simulink model "HEV"  (R2015a)
settings: Solver=ode23tb  StartTime=0.0  StopTime=318  FixedStep=Ts  MaxStep=Ts  RelTol=1  AbsTol=0.5
InitFcn:
  | Ts = 6e-05;   % time step
  | DriveCycleNumber = 1;
  | beginningSim = 1;
undefined symbols (not defined in the file): drive_block, drive_enginemodel, EngineSpeedPower, FuelConsTable, GasEmisTable, h, Hydride, km, magnitude, Metal, Nickel, rad, s, speed, torque
libraries: powerlib x47, driveline x30, simulink x13, simulink_extras x9, electricdrivelib x3, powerlib_extras x3, aerolibconvert2 x2, DC6DriveInternalModels x1
(part 2 of 3)

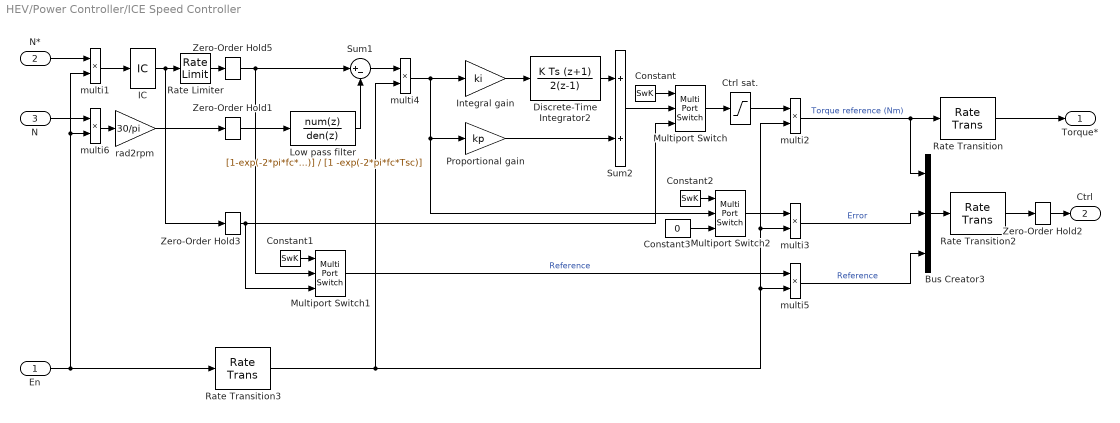
== system HEV/Power Controller/ICE Speed Controller ==
  En : Inport
  N* : Inport  Port=2
  N : Inport  Port=3
  Bus Creator3 : BusCreator  Inputs=3
  Constant : Constant  Value=SwK
  Constant1 : Constant  Value=SwK
  Constant2 : Constant  Value=SwK
  Constant3 : Constant  Value=0
  Ctrl sat. : Saturate  UpperLimit=ctrl_sat(2)  LowerLimit=ctrl_sat(1)
  Discrete-Time Integrator2 : DiscreteIntegrator  IntegratorMethod=Integration: Trapezoidal  SampleTime=Tsc  LimitOutput=on  UpperSaturationLimit=ctrl_sat(2)  LowerSaturationLimit=ctrl_sat(1)
  IC : InitialCondition  Value=0
  Integral gain : Gain  Gain=ki  SaturateOnIntegerOverflow=on  OutDataTypeStr=Inherit: Same as input  ParamDataTypeStr=Inherit: Same as input
  Low pass filter : DiscreteTransferFcn  Numerator=[1-exp(-2*pi*fc*Tsc)]  Denominator=[1 -exp(-2*pi*fc*Tsc)]  SampleTime=Tsc
  Multiport Switch : MultiPortSwitch  Inputs=2  SaturateOnIntegerOverflow=on
  Multiport Switch1 : MultiPortSwitch  Inputs=2  SaturateOnIntegerOverflow=on
  Multiport Switch2 : MultiPortSwitch  Inputs=2  SaturateOnIntegerOverflow=on
  Proportional gain : Gain  Gain=kp  SaturateOnIntegerOverflow=on  OutDataTypeStr=Inherit: Same as input  ParamDataTypeStr=Inherit: Same as input
  Rate Limiter : RateLimiter  RisingSlewLimit=ramp(2)  FallingSlewLimit=ramp(1)  LinearizeAsGain=off
  Rate Transition : RateTransition
  Rate Transition2 : RateTransition
  Rate Transition3 : RateTransition
  Sum1 : Sum  Inputs=|+-  SaturateOnIntegerOverflow=on  InputSameDT=on  OutDataTypeStr=Inherit: Same as first input
  Sum2 : Sum  SaturateOnIntegerOverflow=on  InputSameDT=on  OutDataTypeStr=Inherit: Same as first input
  Zero-Order Hold1 : ZeroOrderHold  SampleTime=Tsc
  Zero-Order Hold2 : ZeroOrderHold  SampleTime=Ts
  Zero-Order Hold3 : ZeroOrderHold  SampleTime=Tsc
  Zero-Order Hold5 : ZeroOrderHold  SampleTime=Tsc
  multi{1..6} (6 alike) : Product
  rad2rpm : Gain  Gain=30/pi  SaturateOnIntegerOverflow=on  OutDataTypeStr=Inherit: Same as input  ParamDataTypeStr=Inherit: Same as input
  Torque* : Outport
  Ctrl : Outport  Port=2
  wires:
  N/1 -> multi6/1
  multi6/1 -> rad2rpm/1
  N*/1 -> multi1/1
  multi1/1 -> IC/1
  Rate Transition3/1 -> multi5/2, multi2/2, multi3/2, multi4/2
  multi4/1 -> Proportional gain/1, Multiport Switch2/2, Integral gain/1
  Low pass filter/1 -> Sum1/2
  multi2/1 -> Bus Creator3/1, Rate Transition/1  "Torque reference (Nm)"
  Multiport Switch1/1 -> multi5/1  "Reference"
  multi5/1 -> Bus Creator3/3  "Reference"
  multi3/1 -> Bus Creator3/2  "Error"
  Multiport Switch2/1 -> multi3/1
  Zero-Order Hold2/1 -> Ctrl/1
  Rate Transition/1 -> Torque*/1
  En/1 -> multi6/2, multi1/2, Rate Transition3/1
  rad2rpm/1 -> Zero-Order Hold1/1
  Constant3/1 -> Multiport Switch2/3
  Constant2/1 -> Multiport Switch2/1
  Zero-Order Hold3/1 -> Multiport Switch1/3, Multiport Switch/3
  Constant1/1 -> Multiport Switch1/1
  Sum2/1 -> Multiport Switch/2
  Constant/1 -> Multiport Switch/1
  Multiport Switch/1 -> Ctrl sat./1
  Zero-Order Hold5/1 -> Multiport Switch1/2, Sum1/1
  Rate Limiter/1 -> Zero-Order Hold5/1
  Bus Creator3/1 -> Rate Transition2/1
  Rate Transition2/1 -> Zero-Order Hold2/1
  Zero-Order Hold1/1 -> Low pass filter/1
  IC/1 -> Zero-Order Hold3/1, Rate Limiter/1
  Proportional gain/1 -> Sum2/2
  Discrete-Time Integrator2/1 -> Sum2/1
  Sum1/1 -> multi4/1
  Integral gain/1 -> Discrete-Time Integrator2/1
  Ctrl sat./1 -> multi2/1

== system HEV/Power Controller/Limit torque ==
  Acceleration : Inport
  Motor Speed (rad/s) : Inport  Port=2
  Abs1 : Abs  SaturateOnIntegerOverflow=on
  Clock1 : Clock
  Compare To Constant : simulink/Logic and Bit Operations/Compare To Constant  relop=>  const=0.05  OutDataTypeStr=uint8  ZeroCross=off
  Gain : Gain  Gain=-1
  Max Torque : Gain  Gain=400
  Product : Product  RndMeth=Zero
  Saturation Dynamic : simulink/Discontinuities/Saturation Dynamic  OutMin=[]  OutMax=[]  OutDataTypeStr=Inherit: Same as second input  OutDataType=sfix(16)  OutScaling=2^-10  DoSatur=off
  Torque vs speed : Lookup  InputValues=[0 1200 2000 3000 4000 5000 6000]*pi/30  Table=[400 400 225 150 100 80 70]  LookUpMeth=Interpolation-Use End Values
  torque : Outport
  wires:
  Motor Speed (rad/s)/1 -> Abs1/1
  Abs1/1 -> Torque vs speed/1
  Max Torque/1 -> Saturation Dynamic/2
  Torque vs speed/1 -> Gain/1, Saturation Dynamic/1
  Clock1/1 -> Compare To Constant/1
  Saturation Dynamic/1 -> Product/1
  Compare To Constant/1 -> Product/2
  Product/1 -> torque/1
  Gain/1 -> Saturation Dynamic/3
  Acceleration/1 -> Max Torque/1

== system HEV/Electric Motor Controller /DC//DC Converter/Bus DC controller ==
  Ubus : Inport
  Uref : Inport  Port=2
  Current controller DISCRETE1 : Subsystem  mask(PI controller){Kp=0.001, Ki=1, Ts=Ts}
      mask prompts: Kp "Proportional gain (Kp)"; Ki "Integral gain (Ki)"; Ts "Sample time (s) :"
      mask help: Proportional-Integral Speed Controller
      mask Display: plot(0,0,100,100,[35,35,65],[70,30,30],[35,65],[45,60])
  Display : Display
      settings: Decimation=100
  Duty Cycles : Subsystem
  Mux : Mux  Inputs=2
  Unit Delay2 : UnitDelay  InitialCondition=.5  SampleTime=Ts
  Zero-Order Hold1 : ZeroOrderHold  SampleTime=Ts
  Duty cycle : Outport  InitialOutput=0
  tag scope: V_DCDC=global
  wires:
  Ubus/1 -> Mux/2, Zero-Order Hold1/1
  Mux/1 -> [V_DCDC]
  Uref/1 -> Current controller DISCRETE1/2(Uref), Mux/1
  Current controller DISCRETE1/1(Ec) -> Duty Cycles/1(Ec)
  Zero-Order Hold1/1 -> Display/1, Current controller DISCRETE1/1(UBus)
  Duty Cycles/1(dc) -> Unit Delay2/1
  Unit Delay2/1 -> Duty cycle/1

== system HEV/Electric Motor Controller /DC//DC Converter/DC//DC converter ==
  Duty Cycle : Inport
  CBus : powerlib/Elements/Series RLC Branch  LConnTagsString=__new0  RConnTagsString=__new0  BranchType=RC  Resistance=0.2  Inductance=1e-3  SetiL0=off  InitialCurrent=0  Capacitance=1130e-6  Setx0=on  InitialVoltage=500  Measurements=None
  CBus1 : powerlib/Elements/Series RLC Branch  LConnTagsString=__new0  RConnTagsString=__new0  BranchType=C  Resistance=0.2  Inductance=1e-3  SetiL0=off  InitialCurrent=0  Capacitance=282e-6  Setx0=on  InitialVoltage=150  Measurements=None
  Chopper : DC6DriveInternalModels/Chopper (average model)  SnubberResistance=10e3  SnubberCapacitance=inf  Ron=1e-3  ForwardVoltages=[1.3,1.3]  IGBTParameters=[0,0]  converterType=Inverter
  L : powerlib/Elements/Series RLC Branch  LConnTagsString=__new0  RConnTagsString=__new0  BranchType=L  Resistance=0.3  Inductance=373e-6  SetiL0=off  InitialCurrent=100  Capacitance=100e-6  Setx0=off  InitialVoltage=0  Measurements=None
  Neutral2 : powerlib/Elements/Neutral  LConnTagsString=a  NodeNumber=10
  V1 : powerlib/Measurements/Voltage Measurement  PhasorSimulation=off  OutputType=Complex  PSBequivalent=0
  + : PMIOPort  Tag=PMCPort  Port=1  Side=Left
  - : PMIOPort  Tag=PMCPort  Port=2  Side=Left
  + bat. : PMIOPort  Tag=PMCPort  Port=3  Side=Right
  - bat. : PMIOPort  Tag=PMCPort  Port=4  Side=Right
  UBus : Outport
  wires:
  Duty Cycle/1 -> Chopper/1
  V1/1 -> UBus/1
  connections:
  Chopper/RConn1 -- L/RConn1
  L/LConn1 -- + bat./RConn1 -- CBus1/LConn1
  CBus1/RConn1 -- - bat./RConn1 -- Chopper/LConn2 -- -/RConn1 -- CBus/RConn1 -- V1/LConn2 -- Neutral2/LConn1
  +/RConn1 -- CBus/LConn1 -- Chopper/LConn1 -- V1/LConn1

== system HEV/Electric Motor Controller /Generator 30kW/Mux ==
  sig* : Inport
  m : Inport  Port=2
  Bus Creator : BusCreator  Inputs=2
  Ctrl : Outport
  wires:
  m/1 -> Bus Creator/2  "m"
  sig*/1 -> Bus Creator/1  "Signals*"
  Bus Creator/1 -> Ctrl/1

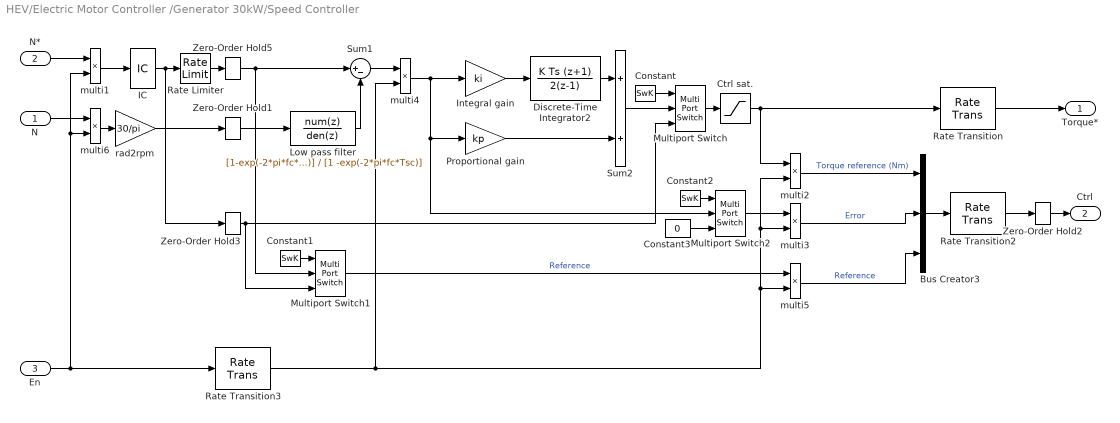
== system HEV/Electric Motor Controller /Generator 30kW/Speed Controller ==
  N : Inport
  N* : Inport  Port=2
  En : Inport  Port=3
  Bus Creator3 : BusCreator  Inputs=3
  Constant : Constant  Value=SwK
  Constant1 : Constant  Value=SwK
  Constant2 : Constant  Value=SwK
  Constant3 : Constant  Value=0
  Ctrl sat. : Saturate  UpperLimit=ctrl_sat(2)  LowerLimit=ctrl_sat(1)
  Discrete-Time Integrator2 : DiscreteIntegrator  IntegratorMethod=Integration: Trapezoidal  SampleTime=Tsc  LimitOutput=on  UpperSaturationLimit=ctrl_sat(2)  LowerSaturationLimit=ctrl_sat(1)
  IC : InitialCondition  Value=0
  Integral gain : Gain  Gain=ki  SaturateOnIntegerOverflow=on  OutDataTypeStr=Inherit: Same as input  ParamDataTypeStr=Inherit: Same as input
  Low pass filter : DiscreteTransferFcn  Numerator=[1-exp(-2*pi*fc*Tsc)]  Denominator=[1 -exp(-2*pi*fc*Tsc)]  SampleTime=Tsc
  Multiport Switch : MultiPortSwitch  Inputs=2  SaturateOnIntegerOverflow=on
  Multiport Switch1 : MultiPortSwitch  Inputs=2  SaturateOnIntegerOverflow=on
  Multiport Switch2 : MultiPortSwitch  Inputs=2  SaturateOnIntegerOverflow=on
  Proportional gain : Gain  Gain=kp  SaturateOnIntegerOverflow=on  OutDataTypeStr=Inherit: Same as input  ParamDataTypeStr=Inherit: Same as input
  Rate Limiter : RateLimiter  RisingSlewLimit=ramp(2)  FallingSlewLimit=ramp(1)  LinearizeAsGain=off
  Rate Transition : RateTransition
  Rate Transition2 : RateTransition
  Rate Transition3 : RateTransition
  Sum1 : Sum  Inputs=|+-  SaturateOnIntegerOverflow=on  InputSameDT=on  OutDataTypeStr=Inherit: Same as first input
  Sum2 : Sum  SaturateOnIntegerOverflow=on  InputSameDT=on  OutDataTypeStr=Inherit: Same as first input
  Zero-Order Hold1 : ZeroOrderHold  SampleTime=Tsc
  Zero-Order Hold2 : ZeroOrderHold  SampleTime=Ts
  Zero-Order Hold3 : ZeroOrderHold  SampleTime=Tsc
  Zero-Order Hold5 : ZeroOrderHold  SampleTime=Tsc
  multi{1..6} (6 alike) : Product
  rad2rpm : Gain  Gain=30/pi  SaturateOnIntegerOverflow=on  OutDataTypeStr=Inherit: Same as input  ParamDataTypeStr=Inherit: Same as input
  Torque* : Outport
  Ctrl : Outport  Port=2
  wires:
  N/1 -> multi6/1
  multi6/1 -> rad2rpm/1
  N*/1 -> multi1/1
  multi1/1 -> IC/1
  Rate Transition3/1 -> multi5/2, multi2/2, multi3/2, multi4/2
  multi4/1 -> Multiport Switch2/2, Proportional gain/1, Integral gain/1
  Low pass filter/1 -> Sum1/2
  multi2/1 -> Bus Creator3/1  "Torque reference (Nm)"
  Multiport Switch1/1 -> multi5/1  "Reference"
  multi5/1 -> Bus Creator3/3  "Reference"
  multi3/1 -> Bus Creator3/2  "Error"
  Multiport Switch2/1 -> multi3/1
  Zero-Order Hold2/1 -> Ctrl/1
  Rate Transition/1 -> Torque*/1
  En/1 -> multi6/2, multi1/2, Rate Transition3/1
  rad2rpm/1 -> Zero-Order Hold1/1
  Constant3/1 -> Multiport Switch2/3
  Constant2/1 -> Multiport Switch2/1
  Zero-Order Hold3/1 -> Multiport Switch1/3, Multiport Switch/3
  Constant1/1 -> Multiport Switch1/1
  Sum2/1 -> Multiport Switch/2
  Constant/1 -> Multiport Switch/1
  Multiport Switch/1 -> Ctrl sat./1
  Zero-Order Hold5/1 -> Multiport Switch1/2, Sum1/1
  Rate Limiter/1 -> Zero-Order Hold5/1
  Bus Creator3/1 -> Rate Transition2/1
  Rate Transition2/1 -> Zero-Order Hold2/1
  Zero-Order Hold1/1 -> Low pass filter/1
  IC/1 -> Zero-Order Hold3/1, Rate Limiter/1
  Proportional gain/1 -> Sum2/2
  Discrete-Time Integrator2/1 -> Sum2/1
  Sum1/1 -> multi4/1
  Integral gain/1 -> Discrete-Time Integrator2/1
  Ctrl sat./1 -> multi2/1, Rate Transition/1

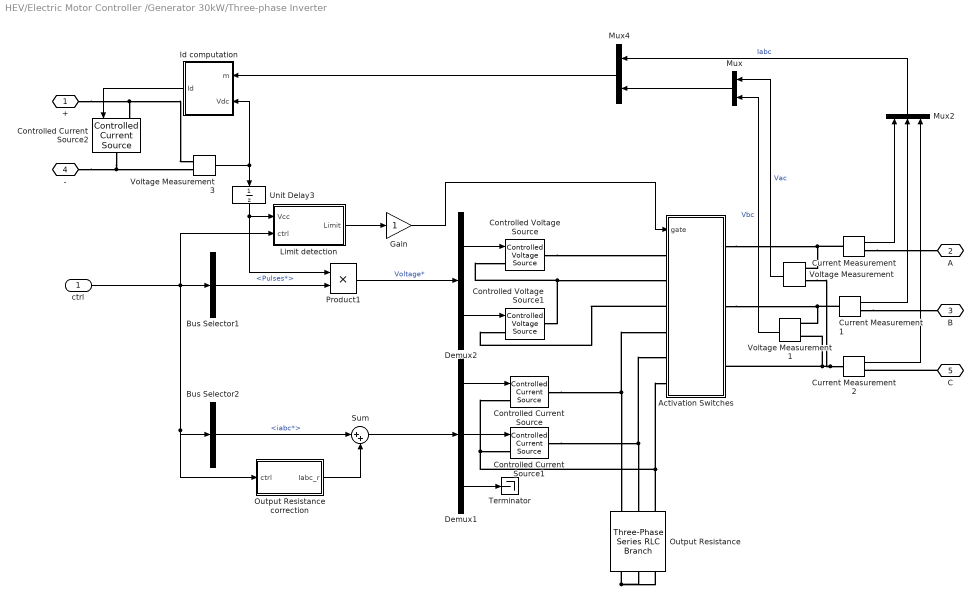
== system HEV/Electric Motor Controller /Generator 30kW/Three-phase Inverter ==
  ctrl : Inport
  Activation Switches : Subsystem
  Bus Selector1 : BusSelector  OutputSignals=Signals*.Pulses*
  Bus Selector2 : BusSelector  OutputSignals=Signals*.iabc*
  Controlled Current Source : powerlib/Electrical Sources/Controlled Current Source  Initialize=on  Source_Type=AC  Amplitude=0  Phase=0  Frequency=0  Measurements=None
  Controlled Current Source1 : powerlib/Electrical Sources/Controlled Current Source  Initialize=on  Source_Type=AC  Amplitude=0  Phase=0  Frequency=0  Measurements=None
  Controlled Current Source2 : powerlib/Electrical Sources/Controlled Current Source  Initialize=on  Source_Type=AC  Amplitude=0  Phase=0  Frequency=0  Measurements=None
  Controlled Voltage Source : powerlib/Electrical Sources/Controlled Voltage Source  Initialize=on  Source_Type=AC  Amplitude=0  Phase=0  Frequency=0  Measurements=None
  Controlled Voltage Source1 : powerlib/Electrical Sources/Controlled Voltage Source  Initialize=on  Source_Type=AC  Amplitude=0  Phase=0  Frequency=0  Measurements=None
  Current Measurement : powerlib/Measurements/Current Measurement  PhasorSimulation=off  OutputType=Complex  PSBequivalent=0
  Current Measurement1 : powerlib/Measurements/Current Measurement  PhasorSimulation=off  OutputType=Complex  PSBequivalent=0
  Current Measurement2 : powerlib/Measurements/Current Measurement  PhasorSimulation=off  OutputType=Complex  PSBequivalent=0
  Demux1 : Demux  Outputs=3
  Demux2 : Demux  Outputs=2
  Gain : Gain
  Id computation : Subsystem
  Limit detection : Subsystem
  Mux : Mux  Inputs=2
  Mux2 : Mux  Inputs=3
  Mux4 : Mux  Inputs=2
  Output Resistance : powerlib/Elements/Three-Phase Series RLC Branch  LConnTagsString=A|B|C  RConnTagsString=A|B|C  BranchType=R  Resistance=100*Resistance  Inductance=1e-3  Capacitance=1e-6  Measurements=Branch voltages and currents
  Output Resistance correction : Subsystem
  Product1 : Product  RndMeth=Zero
  Sum : Sum  Inputs=|++
  Terminator : Terminator
  Unit Delay3 : UnitDelay  SampleTime=Ts
  Voltage Measurement : powerlib/Measurements/Voltage Measurement  PhasorSimulation=off  OutputType=Complex  PSBequivalent=0
  Voltage Measurement1 : powerlib/Measurements/Voltage Measurement  PhasorSimulation=off  OutputType=Complex  PSBequivalent=0
  Voltage Measurement3 : powerlib/Measurements/Voltage Measurement  PhasorSimulation=off  OutputType=Complex  PSBequivalent=0
  + : PMIOPort  Port=1  Side=Right
  A : PMIOPort  Port=2  Side=Left
  B : PMIOPort  Port=3  Side=Left
  - : PMIOPort  Port=4  Side=Right
  C : PMIOPort  Port=5  Side=Left
  wires:
  Gain/1 -> Activation Switches/1(gate)
  Output Resistance correction/1("Iabc_r ") -> Sum/2
  Product1/1 -> Demux2/1  "Voltage*"
  ctrl/1 -> Output Resistance correction/1(ctrl), Bus Selector2/1, Limit detection/2(ctrl), Bus Selector1/1
  Unit Delay3/1 -> Limit detection/1(Vcc), Product1/1
  Sum/1 -> Demux1/1
  Limit detection/1(Limit) -> Gain/1
  Bus Selector2/1 -> Sum/1  "<iabc*>"
  Demux2/1 -> Controlled Voltage Source/1
  Demux2/2 -> Controlled Voltage Source1/1
  Demux1/3 -> Terminator/1
  Demux1/2 -> Controlled Current Source1/1
  Demux1/1 -> Controlled Current Source/1
  Bus Selector1/1 -> Product1/2  "<Pulses*>"
  Voltage Measurement3/1 -> Id computation/2(Vdc), Unit Delay3/1
  Id computation/1(Id) -> Controlled Current Source2/1
  Mux2/1 -> Mux4/1  "Iabc"
  Mux4/1 -> Id computation/1(m)
  Current Measurement2/1 -> Mux2/3
  Mux/1 -> Mux4/2
  Voltage Measurement1/1 -> Mux/2  "Vbc"
  Voltage Measurement/1 -> Mux/1  "Vac"
  Current Measurement1/1 -> Mux2/2
  Current Measurement/1 -> Mux2/1
  connections:
  Activation Switches/LConn3 -- Controlled Voltage Source1/LConn1
  Controlled Voltage Source/RConn1 -- Activation Switches/LConn1
  C/RConn1 -- Current Measurement2/RConn1
  Current Measurement1/RConn1 -- B/RConn1
  Current Measurement/RConn1 -- A/RConn1
  Current Measurement1/LConn1 -- Activation Switches/RConn2 -- Voltage Measurement1/LConn1
  Controlled Voltage Source1/RConn1 -- Activation Switches/LConn2 -- Controlled Voltage Source/LConn1
  Current Measurement2/LConn1 -- Voltage Measurement1/LConn2 -- Activation Switches/RConn3 -- Voltage Measurement/LConn2
  Controlled Current Source1/RConn1 -- Activation Switches/LConn5 -- Output Resistance/LConn2
  Controlled Current Source/RConn1 -- Activation Switches/LConn4 -- Output Resistance/LConn1
  Current Measurement/LConn1 -- Activation Switches/RConn1 -- Voltage Measurement/LConn1
  Output Resistance/RConn1 -- Output Resistance/RConn2 -- Output Resistance/RConn3
  Output Resistance/LConn3 -- Controlled Current Source1/LConn1 -- Controlled Current Source/LConn1 -- Activation Switches/LConn6
  -/RConn1 -- Controlled Current Source2/RConn1 -- Voltage Measurement3/LConn2
  +/RConn1 -- Controlled Current Source2/LConn1 -- Voltage Measurement3/LConn1

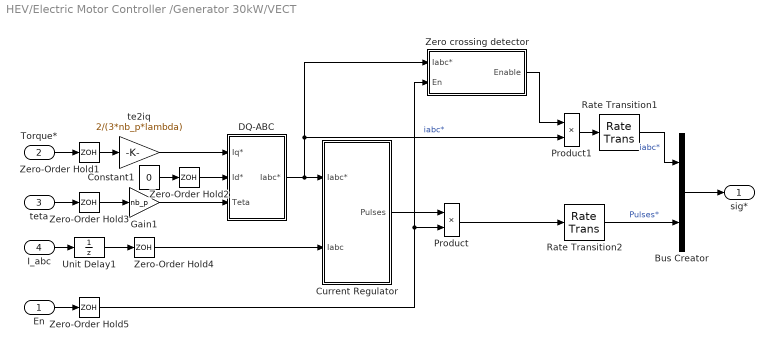
== system HEV/Electric Motor Controller /Generator 30kW/VECT ==
  En : Inport
  Torque* : Inport  Port=2
  teta : Inport  Port=3
  I_abc : Inport  Port=4
  Bus Creator : BusCreator  Inputs=2
  Constant1 : Constant  Value=0
  Current Regulator : Subsystem
  DQ-ABC : Subsystem
  Gain1 : Gain  Gain=nb_p  SaturateOnIntegerOverflow=on  OutDataTypeStr=Inherit: Same as input  ParamDataTypeStr=Inherit: Same as input
  Product : Product  RndMeth=Zero
  Product1 : Product  RndMeth=Zero
  Rate Transition1 : RateTransition
  Rate Transition2 : RateTransition
  Unit Delay1 : UnitDelay  SampleTime=Ts
  Zero crossing detector : Subsystem
  Zero-Order Hold{1..5} (5 alike) : ZeroOrderHold  SampleTime=Ts_vect
  te2iq : Gain  Gain=2/(3*nb_p*lambda)  SaturateOnIntegerOverflow=on  OutDataTypeStr=Inherit: Same as input  ParamDataTypeStr=Inherit: Same as input
  sig* : Outport
  wires:
  Zero-Order Hold5/1 -> Zero crossing detector/2(En), Product/2
  Zero crossing detector/1(Enable) -> Product1/1
  En/1 -> Zero-Order Hold5/1
  Product1/1 -> Rate Transition1/1
  Product/1 -> Rate Transition2/1
  Current Regulator/1(Pulses) -> Product/1
  Zero-Order Hold4/1 -> Current Regulator/2(Iabc)
  Rate Transition1/1 -> Bus Creator/1  "iabc*"
  Rate Transition2/1 -> Bus Creator/2  "Pulses*"
  Bus Creator/1 -> sig*/1
  te2iq/1 -> DQ-ABC/1("Iq* ")
  Zero-Order Hold2/1 -> DQ-ABC/2("Id* ")
  Zero-Order Hold1/1 -> te2iq/1
  teta/1 -> Zero-Order Hold3/1
  Zero-Order Hold3/1 -> Gain1/1
  Torque*/1 -> Zero-Order Hold1/1
  Constant1/1 -> Zero-Order Hold2/1
  Gain1/1 -> DQ-ABC/3(Teta)
  Unit Delay1/1 -> Zero-Order Hold4/1
  DQ-ABC/1(Iabc*) -> Zero crossing detector/1(Iabc*), Product1/2, Current Regulator/1(Iabc*)  "iabc*"
  I_abc/1 -> Unit Delay1/1

== system HEV/Electric Motor Controller /Motor 50kW/Mux ==
  sig : Inport
  m : Inport  Port=2
  Bus Creator : BusCreator  Inputs=2
  Ctrl : Outport
  wires:
  Bus Creator/1 -> Ctrl/1
  sig/1 -> Bus Creator/1  "sig"
  m/1 -> Bus Creator/2  "m"

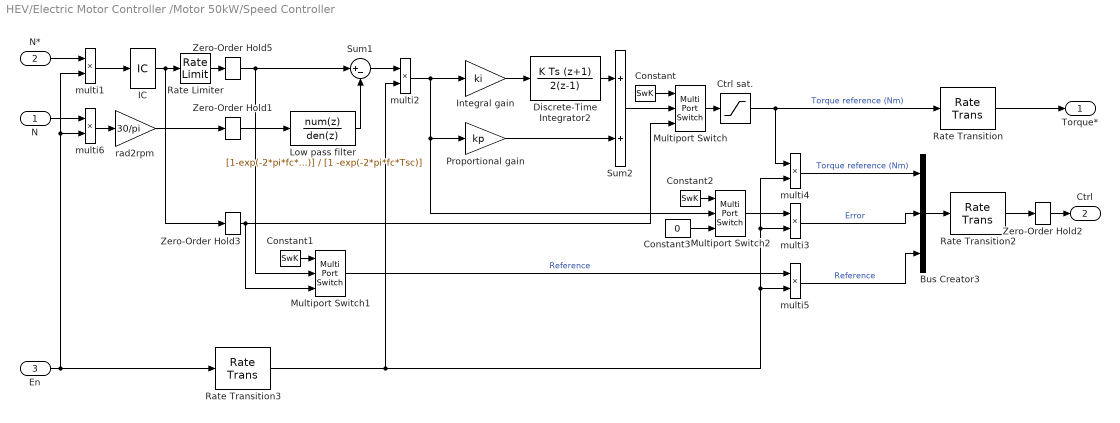
== system HEV/Electric Motor Controller /Motor 50kW/Speed Controller ==
  N : Inport
  N* : Inport  Port=2
  En : Inport  Port=3
  Bus Creator3 : BusCreator  Inputs=3
  Constant : Constant  Value=SwK
  Constant1 : Constant  Value=SwK
  Constant2 : Constant  Value=SwK
  Constant3 : Constant  Value=0
  Ctrl sat. : Saturate  UpperLimit=ctrl_sat(2)  LowerLimit=ctrl_sat(1)
  Discrete-Time Integrator2 : DiscreteIntegrator  IntegratorMethod=Integration: Trapezoidal  SampleTime=Tsc  LimitOutput=on  UpperSaturationLimit=ctrl_sat(2)  LowerSaturationLimit=ctrl_sat(1)
  IC : InitialCondition  Value=0
  Integral gain : Gain  Gain=ki  SaturateOnIntegerOverflow=on  OutDataTypeStr=Inherit: Same as input  ParamDataTypeStr=Inherit: Same as input
  Low pass filter : DiscreteTransferFcn  Numerator=[1-exp(-2*pi*fc*Tsc)]  Denominator=[1 -exp(-2*pi*fc*Tsc)]  SampleTime=Tsc
  Multiport Switch : MultiPortSwitch  Inputs=2  SaturateOnIntegerOverflow=on
  Multiport Switch1 : MultiPortSwitch  Inputs=2  SaturateOnIntegerOverflow=on
  Multiport Switch2 : MultiPortSwitch  Inputs=2  SaturateOnIntegerOverflow=on
  Proportional gain : Gain  Gain=kp  SaturateOnIntegerOverflow=on  OutDataTypeStr=Inherit: Same as input  ParamDataTypeStr=Inherit: Same as input
  Rate Limiter : RateLimiter  RisingSlewLimit=ramp(2)  FallingSlewLimit=ramp(1)  LinearizeAsGain=off
  Rate Transition : RateTransition
  Rate Transition2 : RateTransition
  Rate Transition3 : RateTransition
  Sum1 : Sum  Inputs=|+-  SaturateOnIntegerOverflow=on  InputSameDT=on  OutDataTypeStr=Inherit: Same as first input
  Sum2 : Sum  SaturateOnIntegerOverflow=on  InputSameDT=on  OutDataTypeStr=Inherit: Same as first input
  Zero-Order Hold1 : ZeroOrderHold  SampleTime=Tsc
  Zero-Order Hold2 : ZeroOrderHold  SampleTime=Ts
  Zero-Order Hold3 : ZeroOrderHold  SampleTime=Tsc
  Zero-Order Hold5 : ZeroOrderHold  SampleTime=Tsc
  multi{1..6} (6 alike) : Product
  rad2rpm : Gain  Gain=30/pi  SaturateOnIntegerOverflow=on  OutDataTypeStr=Inherit: Same as input  ParamDataTypeStr=Inherit: Same as input
  Torque* : Outport
  Ctrl : Outport  Port=2
  wires:
  Ctrl sat./1 -> multi4/1, Rate Transition/1  "Torque reference (Nm)"
  Integral gain/1 -> Discrete-Time Integrator2/1
  Sum1/1 -> multi2/1
  Discrete-Time Integrator2/1 -> Sum2/1
  Proportional gain/1 -> Sum2/2
  IC/1 -> Rate Limiter/1, Zero-Order Hold3/1
  Zero-Order Hold1/1 -> Low pass filter/1
  Rate Transition2/1 -> Zero-Order Hold2/1
  Bus Creator3/1 -> Rate Transition2/1
  Low pass filter/1 -> Sum1/2
  Rate Limiter/1 -> Zero-Order Hold5/1
  Zero-Order Hold5/1 -> Sum1/1, Multiport Switch1/2
  Multiport Switch/1 -> Ctrl sat./1
  Constant/1 -> Multiport Switch/1
  Sum2/1 -> Multiport Switch/2
  Constant1/1 -> Multiport Switch1/1
  Zero-Order Hold3/1 -> Multiport Switch/3, Multiport Switch1/3
  Constant2/1 -> Multiport Switch2/1
  Constant3/1 -> Multiport Switch2/3
  rad2rpm/1 -> Zero-Order Hold1/1
  En/1 -> Rate Transition3/1, multi1/2, multi6/2
  Rate Transition/1 -> Torque*/1
  Zero-Order Hold2/1 -> Ctrl/1
  Multiport Switch2/1 -> multi3/1
  multi3/1 -> Bus Creator3/2  "Error"
  multi5/1 -> Bus Creator3/3  "Reference"
  Multiport Switch1/1 -> multi5/1  "Reference"
  multi4/1 -> Bus Creator3/1  "Torque reference (Nm)"
  multi2/1 -> Integral gain/1, Proportional gain/1, Multiport Switch2/2
  Rate Transition3/1 -> multi2/2, multi4/2, multi3/2, multi5/2
  multi6/1 -> rad2rpm/1
  multi1/1 -> IC/1
  N*/1 -> multi1/1
  N/1 -> multi6/1

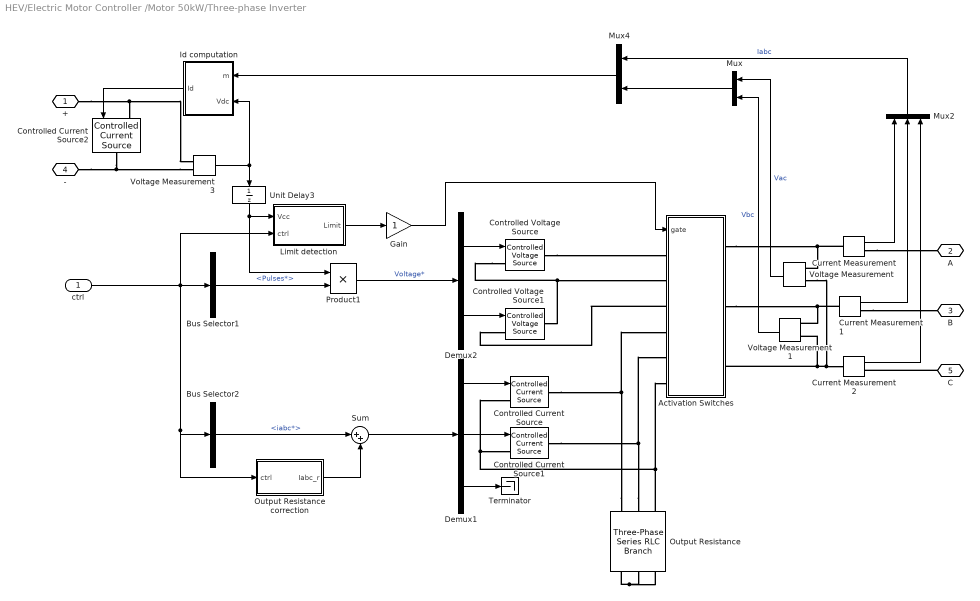
== system HEV/Electric Motor Controller /Motor 50kW/Three-phase Inverter ==
  ctrl : Inport
  Activation Switches : Subsystem
  Bus Selector1 : BusSelector  OutputSignals=sig.Pulses*
  Bus Selector2 : BusSelector  OutputSignals=sig.iabc*
  Controlled Current Source : powerlib/Electrical Sources/Controlled Current Source  Initialize=on  Source_Type=AC  Amplitude=0  Phase=0  Frequency=0  Measurements=None
  Controlled Current Source1 : powerlib/Electrical Sources/Controlled Current Source  Initialize=on  Source_Type=AC  Amplitude=0  Phase=0  Frequency=0  Measurements=None
  Controlled Current Source2 : powerlib/Electrical Sources/Controlled Current Source  Initialize=on  Source_Type=AC  Amplitude=0  Phase=0  Frequency=0  Measurements=None
  Controlled Voltage Source : powerlib/Electrical Sources/Controlled Voltage Source  Initialize=on  Source_Type=AC  Amplitude=0  Phase=0  Frequency=0  Measurements=None
  Controlled Voltage Source1 : powerlib/Electrical Sources/Controlled Voltage Source  Initialize=on  Source_Type=AC  Amplitude=0  Phase=0  Frequency=0  Measurements=None
  Current Measurement : powerlib/Measurements/Current Measurement  PhasorSimulation=off  OutputType=Complex  PSBequivalent=0
  Current Measurement1 : powerlib/Measurements/Current Measurement  PhasorSimulation=off  OutputType=Complex  PSBequivalent=0
  Current Measurement2 : powerlib/Measurements/Current Measurement  PhasorSimulation=off  OutputType=Complex  PSBequivalent=0
  Demux1 : Demux  Outputs=3
  Demux2 : Demux  Outputs=2
  Gain : Gain
  Id computation : Subsystem
  Limit detection : Subsystem
  Mux : Mux  Inputs=2
  Mux2 : Mux  Inputs=3
  Mux4 : Mux  Inputs=2
  Output Resistance : powerlib/Elements/Three-Phase Series RLC Branch  LConnTagsString=A|B|C  RConnTagsString=A|B|C  BranchType=R  Resistance=100*Resistance  Inductance=1e-3  Capacitance=1e-6  Measurements=Branch voltages and currents
  Output Resistance correction : Subsystem
  Product1 : Product  RndMeth=Zero
  Sum : Sum  Inputs=|++
  Terminator : Terminator
  Unit Delay3 : UnitDelay  SampleTime=Ts
  Voltage Measurement : powerlib/Measurements/Voltage Measurement  PhasorSimulation=off  OutputType=Complex  PSBequivalent=0
  Voltage Measurement1 : powerlib/Measurements/Voltage Measurement  PhasorSimulation=off  OutputType=Complex  PSBequivalent=0
  Voltage Measurement3 : powerlib/Measurements/Voltage Measurement  PhasorSimulation=off  OutputType=Complex  PSBequivalent=0
  + : PMIOPort  Port=1  Side=Right
  A : PMIOPort  Port=2  Side=Left
  B : PMIOPort  Port=3  Side=Left
  - : PMIOPort  Port=4  Side=Right
  C : PMIOPort  Port=5  Side=Left
  wires:
  Current Measurement/1 -> Mux2/1
  Current Measurement1/1 -> Mux2/2
  Voltage Measurement/1 -> Mux/1  "Vac"
  Voltage Measurement1/1 -> Mux/2  "Vbc"
  Mux/1 -> Mux4/2
  Current Measurement2/1 -> Mux2/3
  Mux4/1 -> Id computation/1(m)
  Mux2/1 -> Mux4/1  "Iabc"
  Voltage Measurement3/1 -> Unit Delay3/1, Id computation/2(Vdc)
  Bus Selector1/1 -> Product1/2  "<Pulses*>"
  Demux1/1 -> Controlled Current Source/1
  Demux1/2 -> Controlled Current Source1/1
  Demux1/3 -> Terminator/1
  Demux2/2 -> Controlled Voltage Source1/1
  Demux2/1 -> Controlled Voltage Source/1
  Bus Selector2/1 -> Sum/1  "<iabc*>"
  Limit detection/1(Limit) -> Gain/1
  Sum/1 -> Demux1/1
  Unit Delay3/1 -> Product1/1, Limit detection/1(Vcc)
  ctrl/1 -> Bus Selector1/1, Limit detection/2(ctrl), Bus Selector2/1, Output Resistance correction/1(ctrl)
  Product1/1 -> Demux2/1  "Voltage*"
  Gain/1 -> Activation Switches/1(gate)
  Id computation/1(Id) -> Controlled Current Source2/1
  Output Resistance correction/1("Iabc_r ") -> Sum/2
  connections:
  Voltage Measurement3/LConn1 -- Controlled Current Source2/LConn1 -- +/RConn1
  Voltage Measurement3/LConn2 -- Controlled Current Source2/RConn1 -- -/RConn1
  Activation Switches/LConn6 -- Controlled Current Source/LConn1 -- Controlled Current Source1/LConn1 -- Output Resistance/LConn3
  Output Resistance/RConn3 -- Output Resistance/RConn2 -- Output Resistance/RConn1
  Voltage Measurement/LConn1 -- Activation Switches/RConn1 -- Current Measurement/LConn1
  Output Resistance/LConn1 -- Activation Switches/LConn4 -- Controlled Current Source/RConn1
  Output Resistance/LConn2 -- Activation Switches/LConn5 -- Controlled Current Source1/RConn1
  Voltage Measurement/LConn2 -- Activation Switches/RConn3 -- Voltage Measurement1/LConn2 -- Current Measurement2/LConn1
  Controlled Voltage Source/LConn1 -- Activation Switches/LConn2 -- Controlled Voltage Source1/RConn1
  Voltage Measurement1/LConn1 -- Activation Switches/RConn2 -- Current Measurement1/LConn1
  Current Measurement/RConn1 -- A/RConn1
  Current Measurement1/RConn1 -- B/RConn1
  C/RConn1 -- Current Measurement2/RConn1
  Controlled Voltage Source/RConn1 -- Activation Switches/LConn1
  Activation Switches/LConn3 -- Controlled Voltage Source1/LConn1

== system HEV/Electric Motor Controller /Motor 50kW/Torque limitation ==
  N rad/s : Inport
  Torque : Inport  Port=2
  Abs1 : Abs  SaturateOnIntegerOverflow=on
  Gain : Gain  Gain=-1
  Saturation Dynamic : simulink/Discontinuities/Saturation Dynamic  OutMin=[]  OutMax=[]  OutDataTypeStr=Inherit: Same as second input  OutDataType=sfix(16)  OutScaling=2^-10  DoSatur=off
  Torque vs speed profile : Lookup  InputValues=[0 1200 2000 3000 4000 5000 6000]*pi/30  Table=[400 400 225 150 100 80 70]  LookUpMeth=Interpolation-Use End Values
  torque : Outport
  wires:
  N rad/s/1 -> Abs1/1
  Abs1/1 -> Torque vs speed profile/1
  Torque vs speed profile/1 -> Saturation Dynamic/1, Gain/1
  Saturation Dynamic/1 -> torque/1
  Torque/1 -> Saturation Dynamic/2
  Gain/1 -> Saturation Dynamic/3

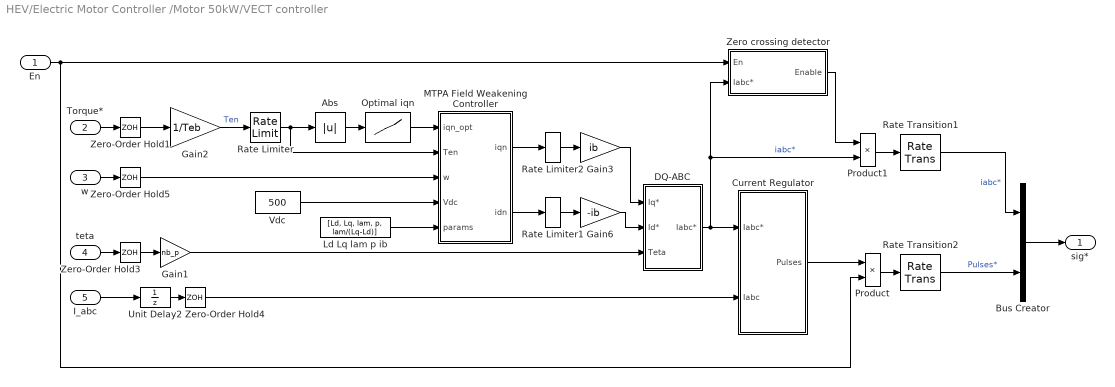
== system HEV/Electric Motor Controller /Motor 50kW/VECT controller ==
  En : Inport
  Torque* : Inport  Port=2
  w : Inport  Port=3
  teta : Inport  Port=4
  I_abc : Inport  Port=5
  Abs : Abs
  Bus Creator : BusCreator  Inputs=2
  Current Regulator : Subsystem
  DQ-ABC : Subsystem
  Gain1 : Gain  Gain=nb_p  SaturateOnIntegerOverflow=on  OutDataTypeStr=Inherit: Same as input  ParamDataTypeStr=Inherit: Same as input
  Gain2 : Gain  Gain=1/Teb  SaturateOnIntegerOverflow=on  OutDataTypeStr=Inherit: Same as input  ParamDataTypeStr=Inherit: Same as input
  Gain3 : Gain  Gain=ib  SaturateOnIntegerOverflow=on  OutDataTypeStr=Inherit: Same as input  ParamDataTypeStr=Inherit: Same as input
  Gain6 : Gain  Gain=-ib  SaturateOnIntegerOverflow=on  OutDataTypeStr=Inherit: Same as input  ParamDataTypeStr=Inherit: Same as input
  Ld Lq lam p ib : Constant  Value=[Ld, Lq, lam, p, lam/(Lq-Ld)]
  MTPA Field Weakening Controller : MATLAB Function  TreatAsAtomicUnit=on  SystemSampleTime=Ts_vect
  Optimal iqn : Lookup  InputValues=ten  Table=iqn
  Product : Product  RndMeth=Zero
  Product1 : Product  RndMeth=Zero
  Rate Limiter : RateLimiter  RisingSlewLimit=10  FallingSlewLimit=-10  LinearizeAsGain=off
  Rate Limiter1 : RateLimiter  RisingSlewLimit=100  FallingSlewLimit=-100  SampleTimeMode=inherited
  Rate Limiter2 : RateLimiter  RisingSlewLimit=100  FallingSlewLimit=-100  SampleTimeMode=inherited
  Rate Transition1 : RateTransition
  Rate Transition2 : RateTransition
  Unit Delay2 : UnitDelay  SampleTime=-1
  Vdc : Constant  Value=500
  Zero crossing detector : Subsystem
  Zero-Order Hold{1,3..5} (4 alike) : ZeroOrderHold  SampleTime=Ts_vect
  sig* : Outport
  wires:
  Unit Delay2/1 -> Zero-Order Hold4/1
  Zero-Order Hold4/1 -> Current Regulator/2(Iabc)
  teta/1 -> Zero-Order Hold3/1
  Zero-Order Hold3/1 -> Gain1/1
  Gain1/1 -> DQ-ABC/3(Teta)
  DQ-ABC/1(Iabc*) -> Current Regulator/1(Iabc*), Zero crossing detector/2(Iabc*), Product1/2  "iabc*"
  I_abc/1 -> Unit Delay2/1
  Torque*/1 -> Zero-Order Hold1/1
  Gain3/1 -> DQ-ABC/1("Iq* ")
  Gain6/1 -> DQ-ABC/2("Id* ")
  Zero-Order Hold1/1 -> Gain2/1
  w/1 -> Zero-Order Hold5/1
  MTPA Field Weakening Controller/2(idn) -> Rate Limiter1/1
  Gain2/1 -> Rate Limiter/1  "Ten"
  Zero-Order Hold5/1 -> MTPA Field Weakening Controller/3(w)
  Ld Lq lam p ib/1 -> MTPA Field Weakening Controller/5(params)
  MTPA Field Weakening Controller/1(iqn) -> Rate Limiter2/1
  Optimal iqn/1 -> MTPA Field Weakening Controller/1(iqn_opt)
  Abs/1 -> Optimal iqn/1
  Vdc/1 -> MTPA Field Weakening Controller/4(Vdc)
  Bus Creator/1 -> sig*/1
  Rate Transition2/1 -> Bus Creator/2  "Pulses*"
  Rate Transition1/1 -> Bus Creator/1  "iabc*"
  Current Regulator/1(Pulses) -> Product/1
  Product/1 -> Rate Transition2/1
  Product1/1 -> Rate Transition1/1
  Zero crossing detector/1(Enable) -> Product1/1
  En/1 -> Zero crossing detector/1(En), Product/2
  Rate Limiter2/1 -> Gain3/1
  Rate Limiter1/1 -> Gain6/1
  Rate Limiter/1 -> Abs/1, MTPA Field Weakening Controller/2(Ten)

== system HEV/Engine Controller/Fuel and Gas Emissions Calculation/Fuel Conversion ==
  Vehicle Speed (km/h) : Inport
  Fuel Consumption (g/s) : Inport  Port=2
  Divide : Product  Inputs=*/
  Gasoline density kg/m^3 : Constant  Value=719.7
  Integrator (total km) : Integrator  InitialCondition=eps
  Integrator (total l) : Integrator  InitialCondition=eps
  Reciprocal : Math  Operator=reciprocal  SaturateOnIntegerOverflow=on
  Saturation : Saturate  UpperLimit=Inf  LowerLimit=0
  Saturation1 : Saturate  UpperLimit=Inf  LowerLimit=0
  Saturation2 : Saturate  UpperLimit=Inf  LowerLimit=0
  Velocity Conversion : aerolibconvert2/Velocity Conversion  IU=km/h  OU=km/s
  g/s to kg/s : Gain  Gain=0.001
  l/km to l/100km : Gain  Gain=100
  liters per km : Product  Inputs=/*
  m^3 to liters : Gain  Gain=1000
  l/100km : Outport
  km/l : Outport  Port=2
  Total Fuel (l) : Outport  Port=3
  wires:
  Vehicle Speed (km/h)/1 -> Velocity Conversion/1
  Velocity Conversion/1 -> Integrator (total km)/1
  Fuel Consumption (g/s)/1 -> g/s to kg/s/1
  g/s to kg/s/1 -> Divide/1
  Gasoline density kg/m^3/1 -> Divide/2
  Divide/1 -> m^3 to liters/1
  m^3 to liters/1 -> Integrator (total l)/1
  Integrator (total km)/1 -> liters per km/1
  Integrator (total l)/1 -> Saturation/1, liters per km/2
  liters per km/1 -> Reciprocal/1, l/km to l/100km/1
  l/km to l/100km/1 -> Saturation2/1
  Reciprocal/1 -> Saturation1/1
  Saturation/1 -> Total Fuel (l)/1
  Saturation1/1 -> km/l/1
  Saturation2/1 -> l/100km/1

== system HEV/Power Controller/Game Theory Controller/Battery Available Power ==
  T ICE : Inport
  P* ICE : Inport  Port=2
  Battery recharge : Inport  Port=3
  ICE speed (rad/s) : Inport  Port=4
  Power limit : Inport  Port=5
  Add2 : Sum  Inputs=-+
  Compare To Zero : simulink/Logic and Bit Operations/Compare To Zero  relop=~=  OutDataTypeStr=boolean
  Gain : Gain  Gain=-1
  Multiplication1 : Product
  Multiplication2 : Product
  Mux2 : Mux  Inputs=2
  Rate Limiter : RateLimiter  RisingSlewLimit=21e3  FallingSlewLimit=-21e3  SampleTimeMode=inherited
  Relay2 : Relay  OnSwitchValue=12e3  OffSwitchValue=11e3
  Saturation Dynamic : simulink/Discontinuities/Saturation Dynamic  OutMin=[]  OutMax=[]  OutDataTypeStr=Inherit: Same as second input  OutDataType=sfix(16)  OutScaling=2^-10  DoSatur=off
  Switch1 : Switch  Criteria=u2 ~= 0
  Switch2 : Switch  Criteria=u2 ~= 0
  Battery power : Outport
  "ICE (P*, P)" : Outport  Port=2
  wires:
  ICE speed (rad/s)/1 -> Multiplication1/2
  Saturation Dynamic/1 -> Battery power/1
  P* ICE/1 -> Add2/2, Multiplication2/1, Relay2/1
  Power limit/1 -> Gain/1, Saturation Dynamic/1
  Gain/1 -> Saturation Dynamic/3
  Mux2/1 -> "ICE (P*, P)"/1
  Relay2/1 -> Multiplication2/2
  Multiplication2/1 -> Mux2/1
  T ICE/1 -> Multiplication1/1
  Multiplication1/1 -> Add2/1, Mux2/2  "P ICE"
  Battery recharge/1 -> Switch1/1, Compare To Zero/1
  Compare To Zero/1 -> Switch1/2, Switch2/2
  Add2/1 -> Switch1/3, Switch2/3  "P batt"
  Switch1/1 -> Rate Limiter/1
  Rate Limiter/1 -> Switch2/1
  Switch2/1 -> Saturation Dynamic/2

== system HEV/Power Controller/Game Theory Controller/Gen torque ==
  T* ICE : Inport
  W gen : Inport  Port=2
  " 1" : Gain  Gain=-1
  " 3" : Gain  Gain=30e3
  " 4" : Gain  Gain=-1/(-2.6-1)
  Abs1 : Abs
  Gen Torque range : simulink/Discontinuities/Saturation Dynamic  OutMin=[]  OutMax=[]  OutDataTypeStr=Inherit: Same as second input  OutDataType=sfix(16)  OutScaling=2^-10  DoSatur=off
  Multiplication2 : Product  Inputs=/
  zero avoider1 : Saturate  UpperLimit=inf  LowerLimit=1
  T* Gen : Outport
  wires:
  T* ICE/1 -> " 4"/1
  Multiplication2/1 -> " 3"/1
  " 3"/1 -> Abs1/1
  W gen/1 -> zero avoider1/1
  Abs1/1 -> Gen Torque range/1, " 1"/1
  " 1"/1 -> Gen Torque range/3
  " 4"/1 -> Gen Torque range/2
  Gen Torque range/1 -> T* Gen/1
  zero avoider1/1 -> Multiplication2/1

== system HEV/Power Controller/Game Theory Controller/Hybrid On//Off ==
  Ref Power : Inport
  Recharge power : Inport  Port=2
  Compare To Zero : simulink/Logic and Bit Operations/Compare To Zero  relop=~=  OutDataTypeStr=boolean
  Compare To Zero1 : simulink/Logic and Bit Operations/Compare To Zero  relop=>  OutDataTypeStr=boolean
  Logical Operator1 : Logic  Operator=OR  AllPortsSameDT=off  OutDataTypeStr=boolean
  Logical Operator2 : Logic  Operator=NOT  AllPortsSameDT=off  OutDataTypeStr=boolean
  Logical Operator3 : Logic  AllPortsSameDT=off  OutDataTypeStr=boolean
  Memory : Memory
  Relay2 : Relay  OnSwitchValue=12e3  OffSwitchValue=11e3  OnOutputValue=0  OffOutputValue=1
  Hybrid : Outport
  wires:
  Relay2/1 -> Logical Operator2/1
  Memory/1 -> Compare To Zero/1
  Logical Operator2/1 -> Logical Operator1/1
  Compare To Zero/1 -> Logical Operator3/2
  Logical Operator3/1 -> Logical Operator1/2
  Compare To Zero1/1 -> Logical Operator3/1
  Ref Power/1 -> Relay2/1, Compare To Zero1/1
  Recharge power/1 -> Memory/1
  Logical Operator1/1 -> Hybrid/1  "Hybrid"

== system HEV/Power Controller/Game Theory Controller/ICE Torque ==
  note: This subsystem is used to calculate the ICE required torque.
      | Also, it calculates the torques needed to stop the ICE when the hybrid mode is off.
  Hybrid : Inport
  W gen : Inport  Port=2
  w* ICE (rpm) : Inport  Port=3
  P* ICE : Inport  Port=4
  w ICE (rad/s) : Inport  Port=5
  ICE Power range : Saturate  UpperLimit=57e3  LowerLimit=-57e3
  Multiplication1 : Product
  Multiplication2 : Product  Inputs=3
  Multiplication3 : Product  Inputs=/*
  Multiplication5 : Product  Inputs=/*
  Rate Limiter2 : RateLimiter  RisingSlewLimit=10  FallingSlewLimit=-10
  Relay1 : Relay  OnSwitchValue=300  OffSwitchValue=200
  Sample & Hold : powerlib_extras/Control  Blocks/Sample & Hold  ic=0
  rpm2rads : Gain  Gain=pi/30
  shed limit : Saturate  UpperLimit=1  LowerLimit=0
  T* ICE : Outport
  wires:
  Relay1/1 -> Rate Limiter2/1
  Hybrid/1 -> Sample & Hold/2
  P* ICE/1 -> ICE Power range/1
  w* ICE (rpm)/1 -> rpm2rads/1
  Multiplication5/1 -> Multiplication1/2  "T* ICE"
  Multiplication1/1 -> Sample & Hold/1
  Multiplication2/1 -> T* ICE/1
  Rate Limiter2/1 -> Multiplication1/1, Multiplication2/1
  ICE Power range/1 -> Multiplication5/2
  rpm2rads/1 -> Multiplication5/1, Multiplication3/1
  w ICE (rad/s)/1 -> Multiplication3/2
  Multiplication3/1 -> shed limit/1  "Loadshed if w < w*"
  Sample & Hold/1 -> Multiplication2/2
  shed limit/1 -> Multiplication2/3
  W gen/1 -> Relay1/1

== system HEV/Electric Motor Controller /DC//DC Converter/Bus DC controller/Current controller DISCRETE1 ==
  UBus : Inport
  Uref : Inport  Port=2
  Clock1 : Clock
  Compare To Constant1 : simulink/Logic and Bit Operations/Compare To Constant  relop=>  const=0.01  OutDataTypeStr=uint8  ZeroCross=off
  Ctrl sat. : Saturate  UpperLimit=0.95  LowerLimit=-0.95
  Discrete-Time Integrator : DiscreteIntegrator  IntegratorMethod=Integration: Trapezoidal  SampleTime=Ts  LimitOutput=on  UpperSaturationLimit=1  LowerSaturationLimit=-1
  Integral gain : Gain  Gain=Ki  SaturateOnIntegerOverflow=on  OutDataTypeStr=Inherit: Same as input  ParamDataTypeStr=Inherit: Same as input
  Product1 : Product  RndMeth=Zero
  Proportional gain : Gain  Gain=Kp  SaturateOnIntegerOverflow=on  OutDataTypeStr=Inherit: Same as input  ParamDataTypeStr=Inherit: Same as input
  Sum1 : Sum  Inputs=+-  SaturateOnIntegerOverflow=on  InputSameDT=on  OutDataTypeStr=Inherit: Same as first input
  Sum2 : Sum  SaturateOnIntegerOverflow=on  InputSameDT=on  OutDataTypeStr=Inherit: Same as first input
  Ec : Outport  InitialOutput=0
  wires:
  Sum2/1 -> Ctrl sat./1
  Discrete-Time Integrator/1 -> Sum2/2
  Uref/1 -> Sum1/2
  UBus/1 -> Sum1/1
  Integral gain/1 -> Discrete-Time Integrator/1
  Proportional gain/1 -> Sum2/1
  Ctrl sat./1 -> Ec/1
  Sum1/1 -> Product1/1
  Clock1/1 -> Compare To Constant1/1
  Compare To Constant1/1 -> Product1/2
  Product1/1 -> Integral gain/1, Proportional gain/1

== system HEV/Electric Motor Controller /DC//DC Converter/Bus DC controller/Duty Cycles ==
  Ec : Inport
  Add : Sum  Inputs=+-
  Bus Creator2 : BusCreator  Inputs=2
  Constant : Constant
  Duty Cycle : Fcn  Expr=0.5*(u[1]+1)
  dc : Outport
  wires:
  Bus Creator2/1 -> dc/1
  Ec/1 -> Duty Cycle/1
  Constant/1 -> Add/1
  Add/1 -> Bus Creator2/2  "IGBT 2"
  Duty Cycle/1 -> Bus Creator2/1, Add/2  "IGBT I"

== system HEV/Electric Motor Controller /Generator 30kW/Three-phase Inverter/Activation Switches ==
  gate : Inport
  Ideal Switch1 : powerlib/Power Electronics/Ideal Switch  Ron=2*Ron  Lon=0  IC=1  Rs=1e6  Cs=inf  Measurements=off
  Ideal Switch2 : powerlib/Power Electronics/Ideal Switch  Ron=2*Ron  Lon=0  IC=1  Rs=1e6  Cs=inf  Measurements=off
  Ideal Switch3 : powerlib/Power Electronics/Ideal Switch  Ron=2*Ron  Lon=0  IC=1  Rs=1e6  Cs=inf  Measurements=off
  Ideal Switch4 : powerlib/Power Electronics/Ideal Switch  Ron=2*Ron  Lon=0  IC=0  Rs=1e6  Cs=inf  Measurements=off
  Ideal Switch5 : powerlib/Power Electronics/Ideal Switch  Ron=2*Ron  Lon=0  IC=0  Rs=1e6  Cs=inf  Measurements=off
  Ideal Switch6 : powerlib/Power Electronics/Ideal Switch  Ron=2*Ron  Lon=0  IC=0  Rs=1e6  Cs=inf  Measurements=off
  Logical Operator : Logic  Operator=NOT  AllPortsSameDT=off  OutDataTypeStr=boolean
  A1 : PMIOPort  Port=1  Side=Left
  a : PMIOPort  Port=2  Side=Right
  B1 : PMIOPort  Port=3  Side=Left
  b : PMIOPort  Port=4  Side=Right
  C1 : PMIOPort  Port=5  Side=Left
  c : PMIOPort  Port=6  Side=Right
  A2 : PMIOPort  Port=7  Side=Left
  B2 : PMIOPort  Port=8  Side=Left
  C2 : PMIOPort  Port=9  Side=Left
  wires:
  Logical Operator/1 -> Ideal Switch6/1, Ideal Switch5/1, Ideal Switch4/1
  gate/1 -> Logical Operator/1, Ideal Switch3/1, Ideal Switch2/1, Ideal Switch1/1
  connections:
  C2/RConn1 -- Ideal Switch6/LConn1
  B2/RConn1 -- Ideal Switch5/LConn1
  A2/RConn1 -- Ideal Switch4/LConn1
  c/RConn1 -- Ideal Switch6/RConn1 -- Ideal Switch3/RConn1
  C1/RConn1 -- Ideal Switch3/LConn1
  b/RConn1 -- Ideal Switch5/RConn1 -- Ideal Switch2/RConn1
  B1/RConn1 -- Ideal Switch2/LConn1
  Ideal Switch4/RConn1 -- a/RConn1 -- Ideal Switch1/RConn1
  A1/RConn1 -- Ideal Switch1/LConn1

== system HEV/Electric Motor Controller /Generator 30kW/Three-phase Inverter/Id computation ==
  m : Inport
  Vdc : Inport  Port=2
  Demux : Subsystem
  Demux1 : Subsystem
  Gain : Gain  Gain=Ron
  Math Function : Math  Operator=magnitude^2  SaturateOnIntegerOverflow=on
  Math Function1 : Math  Operator=magnitude^2  SaturateOnIntegerOverflow=on
  Math Function2 : Math  Operator=magnitude^2  SaturateOnIntegerOverflow=on
  Product1 : Product  Inputs=*/  SaturateOnIntegerOverflow=on  OutDataTypeStr=Inherit: Same as first input
  Sum1 : Sum  Inputs=+++  SaturateOnIntegerOverflow=on
  Sum2 : Sum  Inputs=|++  SaturateOnIntegerOverflow=on
  Sum3 : Sum  SaturateOnIntegerOverflow=on
  Unit Delay1 : UnitDelay  SampleTime=Ts
  Unit Delay4 : UnitDelay  InitialCondition=1  SampleTime=Ts
  Vac x Ia : Product  SaturateOnIntegerOverflow=on  OutDataTypeStr=Inherit: Same as first input
  Vbc x Ib : Product  SaturateOnIntegerOverflow=on  OutDataTypeStr=Inherit: Same as first input
  Zero avoider : Saturate  UpperLimit=inf  LowerLimit=1
  Id : Outport
  wires:
  Zero avoider/1 -> Product1/2
  Product1/1 -> Id/1
  Gain/1 -> Sum2/2
  Demux/3(Vbc) -> Vbc x Ib/1
  Demux/4(Ib) -> Vbc x Ib/2
  Demux/2(Ia) -> Vac x Ia/2
  Demux/1(Vac) -> Vac x Ia/1
  Vdc/1 -> Unit Delay4/1
  Vbc x Ib/1 -> Sum3/2
  Vac x Ia/1 -> Sum3/1
  m/1 -> Demux/1(m), Demux1/1(m)
  Unit Delay1/1 -> Product1/1
  Unit Delay4/1 -> Zero avoider/1
  Demux1/1(Ia) -> Math Function/1
  Demux1/2(Ib) -> Math Function1/1
  Demux1/3(Ic) -> Math Function2/1
  Math Function1/1 -> Sum1/2
  Math Function/1 -> Sum1/1
  Math Function2/1 -> Sum1/3
  Sum1/1 -> Gain/1
  Sum3/1 -> Sum2/1
  Sum2/1 -> Unit Delay1/1

== system HEV/Electric Motor Controller /Generator 30kW/Three-phase Inverter/Limit detection ==
  note: Low pass filter
  note: Low pass filter
  note: Limit = 1 saturation mode (voltage mode)
      | Limit = 0 normal mode (current mode)
  Vcc : Inport
  ctrl : Inport  Port=2
  Bus Selector1 : BusSelector  OutputSignals=m.Stator current is_d (A),m.Stator current is_q (A),m.Rotor speed wm (rad/s)  OutputAsBus=on
  Discrete Transfer Fcn1 : DiscreteTransferFcn  Numerator=[1-exp(-Ts*Fcs*2*pi)]  Denominator=[1 -exp(-Ts*Fcs*2*pi)]  SampleTime=Ts
  Discrete Transfer Fcn3 : DiscreteTransferFcn  Numerator=[1-exp(-Ts*Fcs*2*pi)]  Denominator=[1 -exp(-Ts*Fcs*2*pi)]  SampleTime=Ts
  Gain1 : Gain  Gain=0.9  SaturateOnIntegerOverflow=on  OutDataTypeStr=Inherit: Same as input  ParamDataTypeStr=Inherit: Same as input
  "Internal Vcc " : Fcn  Expr=pi/2*sqrt((Resistance*u(1)-Lq*p*u(3)*u(2))^2+(Resistance*u(2)+Ld*p*u(3)*u(1)+Flux*p*u(3))^2)
  Relational Operator : RelationalOperator  Operator=>  OutDataTypeStr=boolean
  Relational Operator2 : RelationalOperator  Operator=<  OutDataTypeStr=boolean
  S-R Flip-Flop : simulink_extras/Flip Flops/S-R Flip-Flop  initial_condition=0
  Terminator : Terminator
  Limit : Outport
  wires:
  S-R Flip-Flop/2 -> Terminator/1
  Discrete Transfer Fcn3/1 -> Relational Operator/2, Gain1/1
  Gain1/1 -> Relational Operator2/2
  Discrete Transfer Fcn1/1 -> Relational Operator2/1, Relational Operator/1
  "Internal Vcc "/1 -> Discrete Transfer Fcn1/1
  Bus Selector1/1 -> "Internal Vcc "/1
  ctrl/1 -> Bus Selector1/1
  S-R Flip-Flop/1 -> Limit/1
  Relational Operator2/1 -> S-R Flip-Flop/2
  Relational Operator/1 -> S-R Flip-Flop/1
  Vcc/1 -> Discrete Transfer Fcn3/1

== system HEV/Electric Motor Controller /Generator 30kW/Three-phase Inverter/Output Resistance correction ==
  note: Vabc
  ctrl : Inport
  1/R : Gain  Gain=1/(100*Resistance)  SaturateOnIntegerOverflow=on  OutDataTypeStr=Inherit: Same as input  ParamDataTypeStr=Inherit: Same as input
  Bus Selector1 : BusSelector  OutputSignals=m.Stator voltage Vs_d (V),m.Stator voltage Vs_q (V),m.Rotor angle thetam (rad)
  Constant : Constant  Value=0
  Discrete Transfer Fcn1 : DiscreteTransferFcn  Numerator=[1-exp(-Ts/.001)]  Denominator=[1 -exp(-Ts/.001)]  SampleTime=Ts
  Discrete Transfer Fcn2 : DiscreteTransferFcn  Numerator=[1-exp(-Ts/.001)]  Denominator=[1 -exp(-Ts/.001)]  SampleTime=Ts
  Fcn : Fcn  Expr=sin(u)
  Fcn1 : Fcn  Expr=cos(u)
  Mux4 : Mux  Inputs=3
  Mux5 : Mux  Inputs=2
  dq0_to_abc Transformation : powerlib_extras/Measurements/dq0_to_abc Transformation
  poles : Gain  Gain=p  SaturateOnIntegerOverflow=on  OutDataTypeStr=Inherit: Same as input  ParamDataTypeStr=Inherit: Same as input
  "Iabc_r " : Outport
  wires:
  poles/1 -> Fcn/1, Fcn1/1
  Bus Selector1/3 -> poles/1  "<Rotor angle thetam (rad)>"
  Discrete Transfer Fcn1/1 -> Mux4/1
  Discrete Transfer Fcn2/1 -> Mux4/2
  dq0_to_abc Transformation/1 -> 1/R/1
  Constant/1 -> Mux4/3
  Mux5/1 -> dq0_to_abc Transformation/2
  Fcn1/1 -> Mux5/2
  Fcn/1 -> Mux5/1
  Mux4/1 -> dq0_to_abc Transformation/1
  ctrl/1 -> Bus Selector1/1
  Bus Selector1/1 -> Discrete Transfer Fcn1/1  "<Stator voltage Vs_d (V)>"
  Bus Selector1/2 -> Discrete Transfer Fcn2/1  "<Stator voltage Vs_q (V)>"
  1/R/1 -> "Iabc_r "/1

== system HEV/Electric Motor Controller /Generator 30kW/VECT/Current Regulator ==
  Iabc* : Inport
  Iabc : Inport  Port=2
  Demux1 : Demux  Outputs=3
  Demux2 : Demux  Outputs=3
  Mux1 : Mux  Inputs=2
  Relay : Relay  OnSwitchValue=0  OffSwitchValue=0
  Relay1 : Relay  OnSwitchValue=0  OffSwitchValue=0
  Relay2 : Relay  OnSwitchValue=0  OffSwitchValue=0
  Sum : Sum  Inputs=-+  SaturateOnIntegerOverflow=on  InputSameDT=on  OutDataTypeStr=Inherit: Same as first input
  Sum1 : Sum  Inputs=-+  SaturateOnIntegerOverflow=on  InputSameDT=on  OutDataTypeStr=Inherit: Same as first input
  Sum2 : Sum  Inputs=-+  SaturateOnIntegerOverflow=on  InputSameDT=on  OutDataTypeStr=Inherit: Same as first input
  Sum3 : Sum  Inputs=+-
  Sum4 : Sum  Inputs=+-
  Pulses : Outport  InitialOutput=0
  wires:
  Sum4/1 -> Mux1/2
  Sum3/1 -> Mux1/1
  Relay2/1 -> Sum4/2
  Relay1/1 -> Sum4/1, Sum3/2
  Relay/1 -> Sum3/1
  Iabc*/1 -> Demux2/1
  Demux2/1 -> Sum/2
  Demux2/2 -> Sum1/2
  Demux2/3 -> Sum2/2
  Demux1/3 -> Sum2/1
  Sum2/1 -> Relay2/1
  Iabc/1 -> Demux1/1
  Mux1/1 -> Pulses/1
  Demux1/2 -> Sum1/1
  Demux1/1 -> Sum/1
  Sum1/1 -> Relay1/1
  Sum/1 -> Relay/1

== system HEV/Electric Motor Controller /Generator 30kW/VECT/DQ-ABC ==
  "Iq* " : Inport
  "Id* " : Inport  Port=2
  Teta : Inport  Port=3
  Fcn : Fcn  Expr=sin(u)
  Fcn1 : Fcn  Expr=cos(u)
  Gain2 : Gain  SaturateOnIntegerOverflow=on  OutDataTypeStr=Inherit: Same as input  ParamDataTypeStr=Inherit: Same as input
  Gain3 : Gain  SaturateOnIntegerOverflow=on  OutDataTypeStr=Inherit: Same as input  ParamDataTypeStr=Inherit: Same as input
  Gain4 : Gain  SaturateOnIntegerOverflow=on  OutDataTypeStr=Inherit: Same as input  ParamDataTypeStr=Inherit: Same as input
  Mux : Mux
  Mux2 : Mux  Inputs=3
  ia : Fcn  Expr=-u[3]*u[2] + u[4]*u[1]
  ib : Fcn  Expr=(-u[1]+1.7320508*u[2])*u[4]*0.5+(u[2]+1.7320508*u[1])*u[3]*0.5
  ic : Sum  Inputs=--  SaturateOnIntegerOverflow=on  InputSameDT=on  OutDataTypeStr=Inherit: Same as first input
  Iabc* : Outport  InitialOutput=0
  wires:
  Fcn/1 -> Mux/2
  Fcn1/1 -> Mux/1
  Mux2/1 -> Iabc*/1
  Mux/1 -> ib/1, ia/1
  Teta/1 -> Fcn1/1, Fcn/1
  "Id* "/1 -> Mux/3
  "Iq* "/1 -> Mux/4
  Gain3/1 -> Mux2/2
  ic/1 -> Gain4/1
  Gain4/1 -> Mux2/3
  Gain2/1 -> Mux2/1
  ia/1 -> Gain2/1, ic/2
  ib/1 -> Gain3/1, ic/1

== system HEV/Electric Motor Controller /Generator 30kW/VECT/Zero crossing detector ==
  Iabc* : Inport
  En : Inport  Port=2
  D Latch : simulink_extras/Flip Flops/D Latch
  D Latch1 : simulink_extras/Flip Flops/D Latch
  D Latch2 : simulink_extras/Flip Flops/D Latch
  Data Type Conversion : DataTypeConversion
  Data Type Conversion2 : DataTypeConversion
  Demux : Demux  Outputs=3
  Hit Crossing : HitCross
  Mux : Mux  Inputs=3
  Terminator : Terminator
  Terminator1 : Terminator
  Terminator2 : Terminator
  Enable : Outport
  wires:
  D Latch2/2 -> Terminator2/1
  D Latch1/2 -> Terminator1/1
  D Latch/2 -> Terminator/1
  Data Type Conversion2/1 -> Enable/1
  Iabc*/1 -> Hit Crossing/1
  En/1 -> Data Type Conversion/1
  Demux/1 -> D Latch/2
  Mux/1 -> Data Type Conversion2/1
  D Latch2/1 -> Mux/3
  D Latch1/1 -> Mux/2
  D Latch/1 -> Mux/1
  Demux/3 -> D Latch2/2
  Demux/2 -> D Latch1/2
  Hit Crossing/1 -> Demux/1
  Data Type Conversion/1 -> D Latch2/1, D Latch1/1, D Latch/1
